simulink model "sim_FullMRE_case5"  (R2023a)
settings: Solver=ode3  StartTime=0.0  StopTime=500  FixedStep=Ts  MaxStep=Ts  RelTol=1e-4
values from neighbouring files (symbols this model uses):
  b0 = 30    [Initial_par.m]    (also in Test_par.m)
  b1 = 11    [Initial_par.m]    (also in Test_par.m)
  c1 = 1/5    (= 0.2)    [Initial_par.m]    (also in Test_par.m = 1)
  c2 = 1/5    (= 0.2)    [Initial_par.m]    (also in Test_par.m = 1)
  c3 = 1/5    (= 0.2)    [Initial_par.m]    (also in Test_par.m = 1)
  gamma = 20    [Initial_par.m]    (also in Test_par.m = 1)
  kpa = [kap1,kap2,kap3]    [Initial_par.m]    (also in Test_par.m)
  N = 3    [Initial_par.m]    (also in Test_par.m)
  p0 = 625    [Initial_par.m]    (also in Test_par.m = 10000)
  p1 = 500    [Initial_par.m]    (also in Test_par.m = 4000)
  p2 = 150    [Initial_par.m]    (also in Test_par.m = 600)
  p3 = 20    [Initial_par.m]    (also in Test_par.m = 40)
  th = [0.1,0.5,1.5]'    [Initial_par.m]    (also in Test_par.m = [0.4,0.5,0.1]')
  Ts = 1e-3    (= 0.001)    [Initial_par.m]    (also in Test_par.m; fig_test_draw.m)
  vari = SD^2    (= 1e-06)    [Initial_par.m]    (also in Test_par.m)
  x0 = [0,0,0]'    [Initial_par.m]    (also in TO_sys.m = x_init; Test_par.m)
  zeta0 = -z0    [Initial_par.m]    (also in Test_par.m)
undefined symbols (not defined in the file or in its folder): Phi0, z0
libraries: matrix_library x5
settings Model: Creator=stt  LastModifiedBy=stt
settings SolverCC: SolverResetMethod=Robust
settings OptimizationCC: ReuseModelBlockBuffer=off

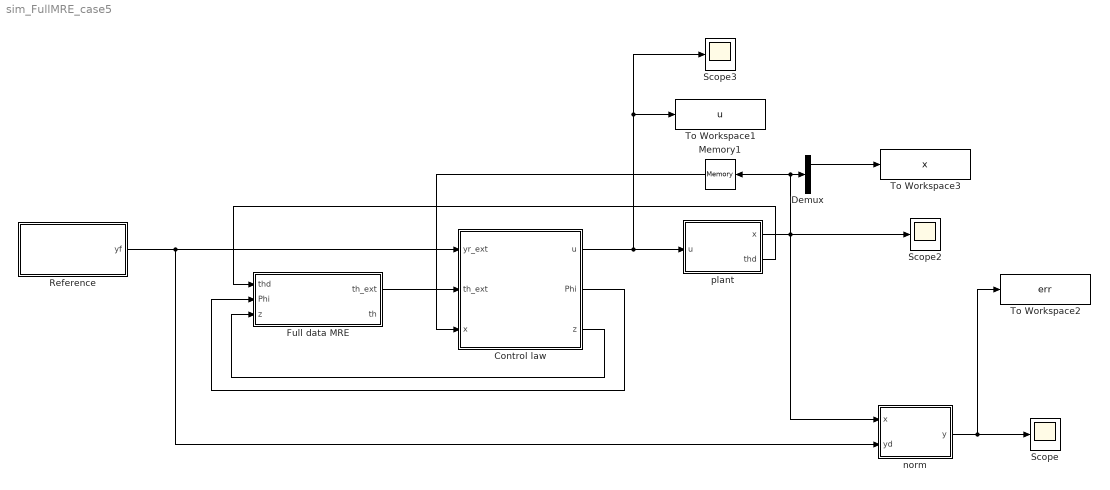
== system sim_FullMRE_case5 ==
  Control law : Subsystem
  Demux : Demux  Outputs=3
  Full data MRE : Subsystem
  Memory1 : Memory  InitialCondition=x0
  Reference : Subsystem
  Scope : Scope
  Scope2 : Scope
  Scope3 : Scope
  To Workspace1 : ToWorkspace  VariableName=u  SaveFormat=Timeseries  SampleTime=-1
  To Workspace2 : ToWorkspace  VariableName=err  SaveFormat=Timeseries  SampleTime=-1
  To Workspace3 : ToWorkspace  VariableName=x  SaveFormat=Timeseries  SampleTime=-1
  norm : MATLAB Function  TreatAsAtomicUnit=on
  plant : Subsystem
  wires:
  norm/1(y) -> To Workspace2/1, Scope/1
  plant/1(x) -> Demux/1, Memory1/1, norm/1(x), Scope2/1
  Demux/1 -> To Workspace3/1
  Control law/2(Phi) -> Full data MRE/2(Phi)
  Control law/1(u) -> To Workspace1/1, Scope3/1, plant/1(u)
  Memory1/1 -> Control law/3(x)
  Full data MRE/1(th_ext) -> Control law/2(th_ext)
  Control law/3(z) -> Full data MRE/3(z)
  plant/2(thd) -> Full data MRE/1(thd)
  Reference/1(yf) -> norm/2(yd), Control law/1(yr_ext)

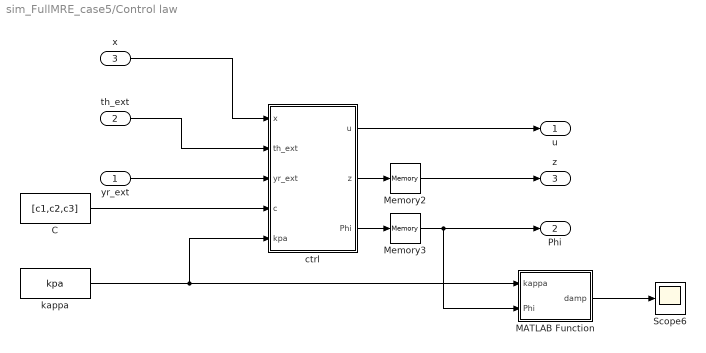
== system sim_FullMRE_case5/Control law ==
  yr_ext : Inport
  th_ext : Inport  Port=2
  x : Inport  Port=3
  C : Constant  Value=[c1,c2,c3]
  MATLAB Function : MATLAB Function  TreatAsAtomicUnit=on
  Memory2 : Memory  InitialCondition=z0
  Memory3 : Memory  InitialCondition=Phi0
  Scope6 : Scope
  ctrl : MATLAB Function  TreatAsAtomicUnit=on
  kappa : Constant  Value=kpa
  u : Outport
  Phi : Outport  Port=2
  z : Outport  Port=3
  wires:
  ctrl/3(Phi) -> Memory3/1
  Memory3/1 -> MATLAB Function/2(Phi), Phi/1
  th_ext/1 -> ctrl/2(th_ext)
  kappa/1 -> ctrl/5(kpa), MATLAB Function/1(kappa)
  C/1 -> ctrl/4(c)
  Memory2/1 -> z/1
  ctrl/2(z) -> Memory2/1
  yr_ext/1 -> ctrl/3(yr_ext)
  x/1 -> ctrl/1(x)
  ctrl/1(u) -> u/1
  MATLAB Function/1(damp) -> Scope6/1

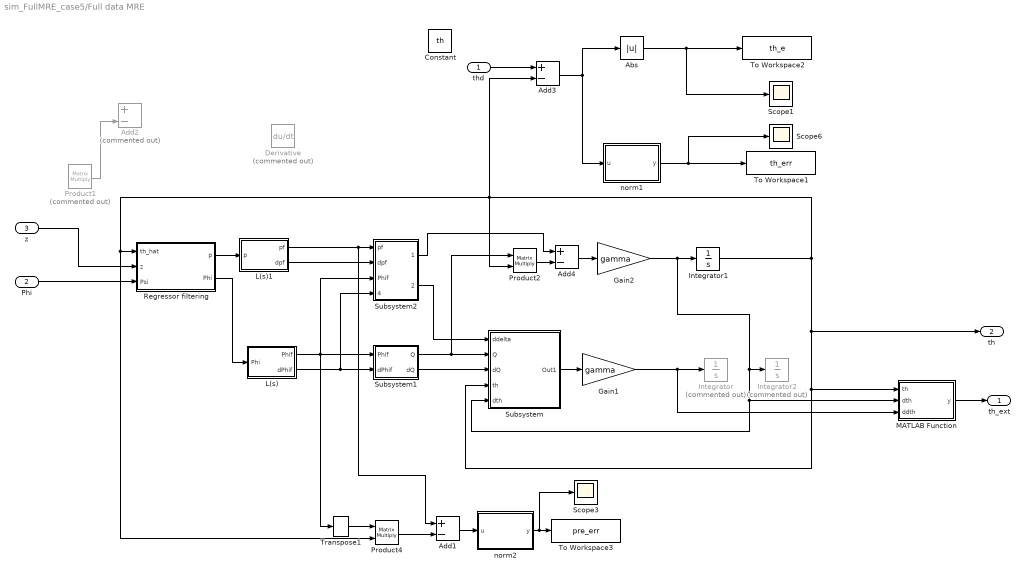
== system sim_FullMRE_case5/Full data MRE ==
  thd : Inport
  Phi : Inport  Port=2
  z : Inport  Port=3
  Abs : Abs  SaturateOnIntegerOverflow=off
  Add1 : Sum  Inputs=+-
  Add2 : Sum  Commented=on  Inputs=+-
  Add3 : Sum  Inputs=+-
  Add4 : Sum  Inputs=+-
  Constant : Constant  Value=th
  Derivative : Derivative  Commented=on
  Gain1 : Gain  Gain=gamma
  Gain2 : Gain  Gain=gamma
  Integrator : Integrator  Commented=on  InitialCondition=zeros(N,1)
  Integrator1 : Integrator  InitialCondition=zeros(N,1)
  Integrator2 : Integrator  Commented=on  InitialCondition=zeros(N,1)
  L(s) : Subsystem
  L(s)1 : Subsystem
  MATLAB Function : MATLAB Function  TreatAsAtomicUnit=on
  Product1 : Product  Commented=on  Multiplication=Matrix(*)
  Product2 : Product  Multiplication=Matrix(*)
  Product4 : Product  Multiplication=Matrix(*)
  Regressor filtering : Subsystem
  Scope1 : Scope
  Scope3 : Scope
  Scope6 : Scope
  Subsystem : Subsystem
  Subsystem1 : Subsystem
  Subsystem2 : Subsystem
  To Workspace1 : ToWorkspace  VariableName=th_err  SaveFormat=Timeseries  SampleTime=-1
  To Workspace2 : ToWorkspace  VariableName=th_e  SaveFormat=Timeseries  SampleTime=-1
  To Workspace3 : ToWorkspace  VariableName=pre_err  SaveFormat=Timeseries  SampleTime=-1
  Transpose1 : matrix_library/Transpose
  norm1 : MATLAB Function  TreatAsAtomicUnit=on
  norm2 : MATLAB Function  TreatAsAtomicUnit=on
  th_ext : Outport
  th : Outport  Port=2
  wires:
  MATLAB Function/1(y) -> th_ext/1
  norm1/1(y) -> To Workspace1/1, Scope6/1
  thd/1 -> Add3/1
  Regressor filtering/2(Phi) -> L(s)/1(Phi)
  Regressor filtering/1(p) -> L(s)1/1(p)
  z/1 -> Regressor filtering/2(z)
  Phi/1 -> Regressor filtering/3(Psi)
  L(s)/1(Phif) -> Subsystem2/3(Phif), Transpose1/1, Subsystem1/1(Phif)
  L(s)/2(dPhif) -> Subsystem2/4(dPhif), Subsystem1/2(dPhif)
  Integrator1/1 -> Subsystem/4(th), MATLAB Function/1(th), th/1, Add3/2, Product2/2, Product4/2, Regressor filtering/1(th_hat)
  L(s)1/2(dpf) -> Subsystem2/2(dpf)
  Subsystem1/1(Q) -> Product2/1, Subsystem/2(Q)
  Add3/1 -> norm1/1(u), Abs/1
  Abs/1 -> To Workspace2/1, Scope1/1
  norm2/1(y) -> Scope3/1, To Workspace3/1
  Add1/1 -> norm2/1(u)
  Product4/1 -> Add1/2
  Transpose1/1 -> Product4/1
  L(s)1/1(pf) -> Add1/1, Subsystem2/1(pf)
  Subsystem/1(Out1) -> Gain1/1
  Product1/1 -> Add2/2
  Subsystem1/2(dQ) -> Subsystem/3(dQ)
  Subsystem2/2(ddelta) -> Subsystem/1(ddelta)
  Gain1/1 -> MATLAB Function/3(ddth), Integrator/1
  Gain2/1 -> Integrator2/1, MATLAB Function/2(dth), Subsystem/5(dth), Integrator1/1
  Product2/1 -> Add4/2
  Subsystem2/1(delta) -> Add4/1
  Add4/1 -> Gain2/1

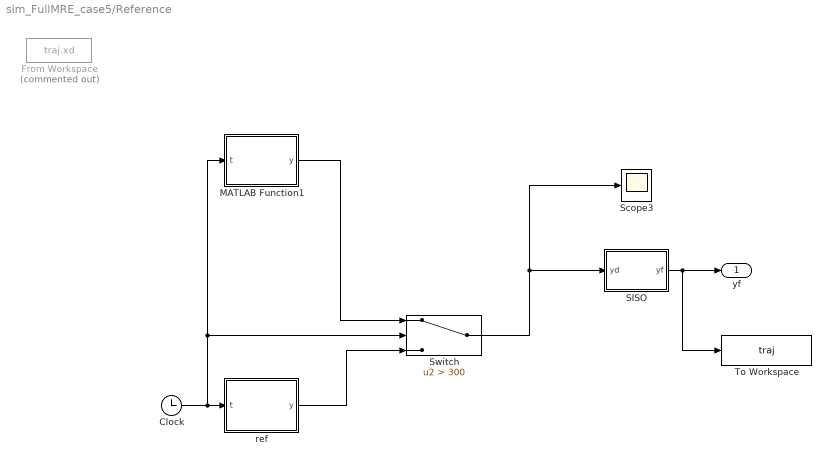
== system sim_FullMRE_case5/Reference ==
  Clock : Clock
  From Workspace : FromWorkspace  Commented=on  VariableName=traj.xd
  MATLAB Function1 : MATLAB Function  TreatAsAtomicUnit=on
  SISO : Subsystem
  Scope3 : Scope
  Switch : Switch  Criteria=u2 > Threshold  Threshold=300  SaturateOnIntegerOverflow=off  InputSameDT=off
  To Workspace : ToWorkspace  VariableName=traj  SaveFormat=Timeseries  SampleTime=-1
  ref : MATLAB Function  TreatAsAtomicUnit=on
  yf : Outport
  wires:
  Switch/1 -> Scope3/1, SISO/1(yd)
  Clock/1 -> MATLAB Function1/1(t), Switch/2, ref/1(t)
  ref/1(y) -> Switch/3
  MATLAB Function1/1(y) -> Switch/1
  SISO/1(yf) -> To Workspace/1, yf/1

== system sim_FullMRE_case5/plant ==
  u : Inport
  Add : Sum
  MATLAB Function : MATLAB Function  TreatAsAtomicUnit=on
  Random Number : RandomNumber  Variance=vari  SampleTime=Ts
  S-Function : S-Function  FunctionName=TO_sys  Parameters=x0,th  SFunctionDeploymentMode=off  EnableBusSupport=off
  x : Outport
  thd : Outport  Port=2
  wires:
  u/1 -> S-Function/1
  S-Function/1 -> MATLAB Function/1(u)
  Add/1 -> x/1
  MATLAB Function/2(thd) -> thd/1
  MATLAB Function/1(x) -> Add/2
  Random Number/1 -> Add/1

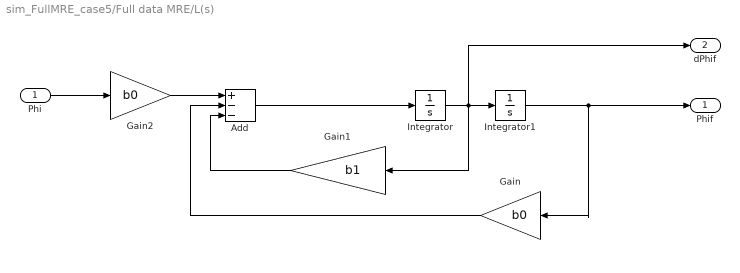
== system sim_FullMRE_case5/Full data MRE/L(s) ==
  Phi : Inport
  Add : Sum  Inputs=+--
  Gain : Gain  Gain=b0
  Gain1 : Gain  Gain=b1
  Gain2 : Gain  Gain=b0
  Integrator : Integrator
  Integrator1 : Integrator
  Phif : Outport
  dPhif : Outport  Port=2
  wires:
  Phi/1 -> Gain2/1
  Integrator1/1 -> Gain/1, Phif/1
  Add/1 -> Integrator/1
  Integrator/1 -> Gain1/1, dPhif/1, Integrator1/1
  Gain1/1 -> Add/3
  Gain/1 -> Add/2
  Gain2/1 -> Add/1

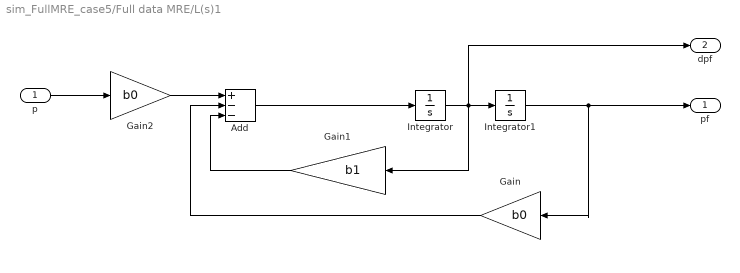
== system sim_FullMRE_case5/Full data MRE/L(s)1 ==
  p : Inport
  Add : Sum  Inputs=+--
  Gain : Gain  Gain=b0
  Gain1 : Gain  Gain=b1
  Gain2 : Gain  Gain=b0
  Integrator : Integrator
  Integrator1 : Integrator
  pf : Outport
  dpf : Outport  Port=2
  wires:
  p/1 -> Gain2/1
  Integrator1/1 -> Gain/1, pf/1
  Add/1 -> Integrator/1
  Integrator/1 -> Gain1/1, dpf/1, Integrator1/1
  Gain1/1 -> Add/3
  Gain/1 -> Add/2
  Gain2/1 -> Add/1

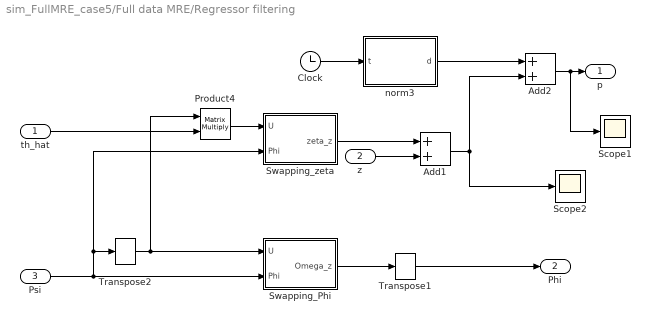
== system sim_FullMRE_case5/Full data MRE/Regressor filtering ==
  th_hat : Inport
  z : Inport  Port=2
  Psi : Inport  Port=3
  Add1 : Sum
  Add2 : Sum
  Clock : Clock
  Product4 : Product  Multiplication=Matrix(*)
  Scope1 : Scope
  Scope2 : Scope
  Swapping_Phi : Subsystem
  Swapping_zeta : Subsystem
  Transpose1 : matrix_library/Transpose
  Transpose2 : matrix_library/Transpose
  norm3 : MATLAB Function  TreatAsAtomicUnit=on
  p : Outport
  Phi : Outport  Port=2
  wires:
  Product4/1 -> Swapping_zeta/1(U)
  th_hat/1 -> Product4/2
  Psi/1 -> Swapping_Phi/2(Phi), Swapping_zeta/2(Phi), Transpose2/1
  Swapping_zeta/1(zeta_z) -> Add1/1
  Transpose2/1 -> Swapping_Phi/1(U), Product4/1
  z/1 -> Add1/2
  Add1/1 -> Add2/2, Scope2/1
  Swapping_Phi/1(Omega_z) -> Transpose1/1
  Transpose1/1 -> Phi/1
  Clock/1 -> norm3/1(t)
  Add2/1 -> Scope1/1, p/1
  norm3/1(d) -> Add2/1

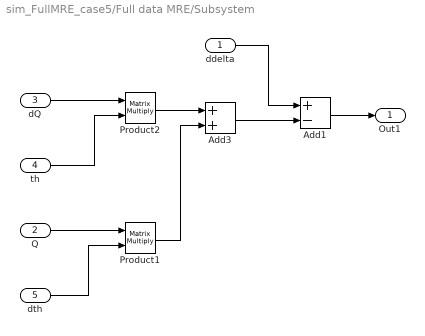
== system sim_FullMRE_case5/Full data MRE/Subsystem ==
  ddelta : Inport
  Q : Inport  Port=2
  dQ : Inport  Port=3
  th : Inport  Port=4
  dth : Inport  Port=5
  Add1 : Sum  Inputs=+-
  Add3 : Sum
  Product1 : Product  Multiplication=Matrix(*)
  Product2 : Product  Multiplication=Matrix(*)
  Out1 : Outport
  wires:
  dQ/1 -> Product2/1
  th/1 -> Product2/2
  Product2/1 -> Add3/1
  Q/1 -> Product1/1
  dth/1 -> Product1/2
  Product1/1 -> Add3/2
  Add3/1 -> Add1/2
  ddelta/1 -> Add1/1
  Add1/1 -> Out1/1

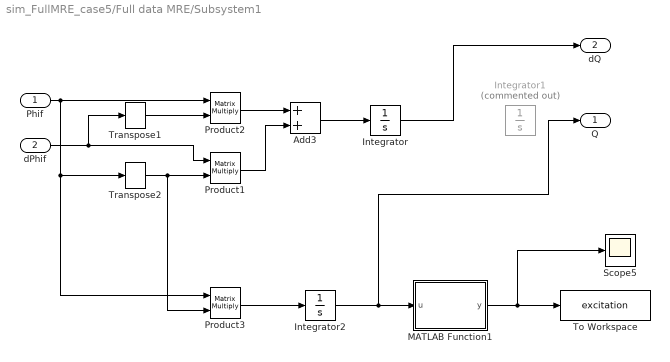
== system sim_FullMRE_case5/Full data MRE/Subsystem1 ==
  Phif : Inport
  dPhif : Inport  Port=2
  Add3 : Sum
  Integrator : Integrator
  Integrator1 : Integrator  Commented=on
  Integrator2 : Integrator
  MATLAB Function1 : MATLAB Function  TreatAsAtomicUnit=on
  Product1 : Product  Multiplication=Matrix(*)
  Product2 : Product  Multiplication=Matrix(*)
  Product3 : Product  Multiplication=Matrix(*)
  Scope5 : Scope
  To Workspace : ToWorkspace  VariableName=excitation  SaveFormat=Timeseries  SampleTime=-1
  Transpose1 : matrix_library/Transpose
  Transpose2 : matrix_library/Transpose
  Q : Outport
  dQ : Outport  Port=2
  wires:
  Phif/1 -> Product2/1, Product3/1, Transpose2/1
  dPhif/1 -> Product1/1, Transpose1/1
  Product1/1 -> Add3/2
  Transpose1/1 -> Product2/2
  Transpose2/1 -> Product3/2, Product1/2
  Product2/1 -> Add3/1
  Add3/1 -> Integrator/1
  Integrator/1 -> dQ/1
  Integrator2/1 -> Q/1, MATLAB Function1/1(u)
  Product3/1 -> Integrator2/1
  MATLAB Function1/1(y) -> Scope5/1, To Workspace/1

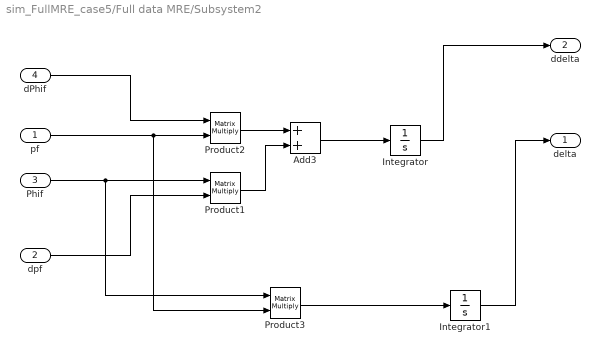
== system sim_FullMRE_case5/Full data MRE/Subsystem2 ==
  pf : Inport
  dpf : Inport  Port=2
  Phif : Inport  Port=3
  dPhif : Inport  Port=4
  Add3 : Sum
  Integrator : Integrator
  Integrator1 : Integrator
  Product1 : Product  Multiplication=Matrix(*)
  Product2 : Product  Multiplication=Matrix(*)
  Product3 : Product  Multiplication=Matrix(*)
  delta : Outport
  ddelta : Outport  Port=2
  wires:
  Product1/1 -> Add3/2
  Product2/1 -> Add3/1
  Integrator/1 -> ddelta/1
  Integrator1/1 -> delta/1
  pf/1 -> Product3/2, Product2/2
  dPhif/1 -> Product2/1
  Phif/1 -> Product3/1, Product1/1
  dpf/1 -> Product1/2
  Add3/1 -> Integrator/1
  Product3/1 -> Integrator1/1

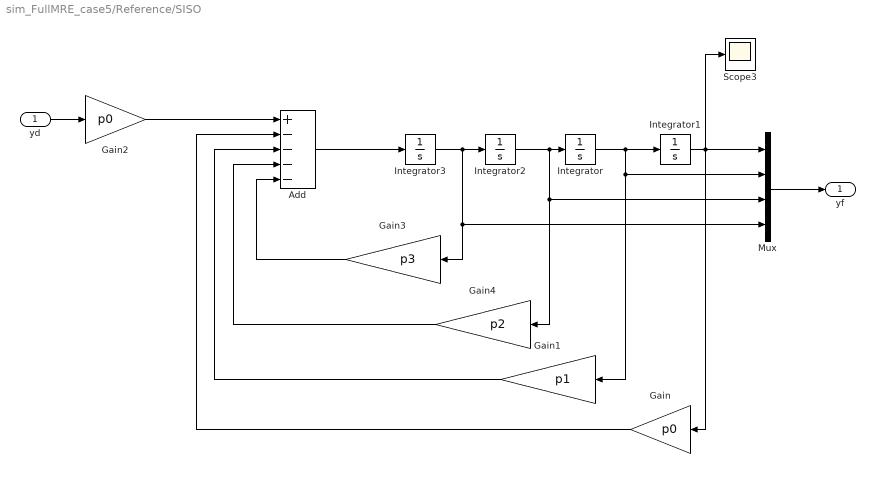
== system sim_FullMRE_case5/Reference/SISO ==
  yd : Inport
  Add : Sum  Inputs=+----
  Gain : Gain  Gain=p0
  Gain1 : Gain  Gain=p1
  Gain2 : Gain  Gain=p0
  Gain3 : Gain  Gain=p3
  Gain4 : Gain  Gain=p2
  Integrator{,1..3} (4 alike) : Integrator
  Mux : Mux
  Scope3 : Scope
  yf : Outport
  wires:
  yd/1 -> Gain2/1
  Add/1 -> Integrator3/1
  Integrator/1 -> Gain1/1, Mux/2, Integrator1/1
  Gain1/1 -> Add/3
  Gain/1 -> Add/2
  Gain2/1 -> Add/1
  Integrator2/1 -> Gain4/1, Mux/3, Integrator/1
  Integrator3/1 -> Gain3/1, Mux/4, Integrator2/1
  Gain3/1 -> Add/5
  Gain4/1 -> Add/4
  Mux/1 -> yf/1
  Integrator1/1 -> Mux/1, Scope3/1, Gain/1

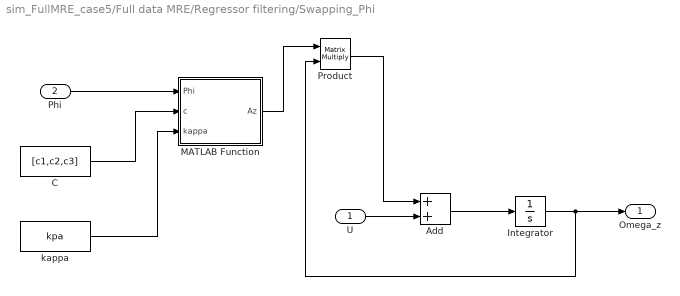
== system sim_FullMRE_case5/Full data MRE/Regressor filtering/Swapping_Phi ==
  U : Inport
  Phi : Inport  Port=2
  Add : Sum
  C : Constant  Value=[c1,c2,c3]
  Integrator : Integrator
  MATLAB Function : MATLAB Function  TreatAsAtomicUnit=on
  Product : Product  Multiplication=Matrix(*)
  kappa : Constant  Value=kpa
  Omega_z : Outport
  wires:
  Phi/1 -> MATLAB Function/1(Phi)
  C/1 -> MATLAB Function/2(c)
  kappa/1 -> MATLAB Function/3(kappa)
  MATLAB Function/1(Az) -> Product/1
  Product/1 -> Add/1
  Add/1 -> Integrator/1
  U/1 -> Add/2
  Integrator/1 -> Product/2, Omega_z/1

== system sim_FullMRE_case5/Full data MRE/Regressor filtering/Swapping_zeta ==
  U : Inport
  Phi : Inport  Port=2
  Add : Sum
  C : Constant  Value=[c1,c2,c3]
  Integrator : Integrator  InitialCondition=zeta0
  MATLAB Function : MATLAB Function  TreatAsAtomicUnit=on
  Product : Product  Multiplication=Matrix(*)
  kappa : Constant  Value=kpa
  zeta_z : Outport
  wires:
  Phi/1 -> MATLAB Function/1(Phi)
  C/1 -> MATLAB Function/2(c)
  kappa/1 -> MATLAB Function/3(kappa)
  MATLAB Function/1(Az) -> Product/1
  Product/1 -> Add/1
  Add/1 -> Integrator/1
  U/1 -> Add/2
  Integrator/1 -> Product/2, zeta_z/1

== matlab function sim_FullMRE_case5/Full data MRE/norm2 ==
  data: u input; y output
function y = fcn(u)

y = norm(u);

== matlab function sim_FullMRE_case5/Control law/MATLAB Function ==
  data: kappa input; damp output; Phi input
function damp = fcn(kappa,Phi)
kap1=kappa(1);kap2=kappa(2);kap3=kappa(3);
phi1=Phi(:,1);phi2=Phi(:,2);phi3=Phi(:,3);
damp=-[kap1*norm(phi1)^2,kap2*norm(phi2)^2,kap3*norm(phi3)^2];

== matlab function sim_FullMRE_case5/Reference/ref ==
  data: t input; y output
function y = fcn(t)


if t<20
    y=0.6;
elseif t<60
    y=0.1;% - 0.4*(tanh((t-30)/5)-1)/2;
elseif t<100
    y=-0.4;% - 0.3*(tanh((t-80)/5)-1)/2;
else
    y=-0.2;
end
% if t<20
%     y=0.5+0.5*(tanh((t-10)/5)-1)/2;
% elseif t<60
%     y=0.3 - 0.2*(tanh((t-40)/5)-1)/2;
% elseif t<120
%     y=-0.2 - 0.5*(tanh((t-90)/5)-1)/2;
% else
%     y=-0.2; %- 0.9*(tanh((t-150)/5)-1)/2;
% end
% y=y*2;
% T=25;
% y=0.5*sin(t*2*pi/T);

% if t>=120
%     y=0;
% end

== matlab function sim_FullMRE_case5/Control law/ctrl ==
  data: x input; th_ext input; yr_ext input; u output; c input; kpa input; z output; Phi output
function [u,z,Phi] = fcn(x,th_ext,yr_ext,c,kpa)



[alpha1,alpha2,u,z,Phi]=virtual_ctrl(x,th_ext,yr_ext,kpa,c);
vir_u=[alpha1,alpha2];

== matlab function sim_FullMRE_case5/Full data MRE/Subsystem1/MATLAB Function1 ==
  data: u input; y output
function y = fcn(u)

y = min(svd(u));

== matlab function sim_FullMRE_case5/Reference/MATLAB Function1 ==
  data: y output; t input
function y = fcn(t)

T=25;

if t<300
    
    y=-0.2;
elseif t<400
    y=-0.2+0.1*sin((t-300)*2*pi/T);
else
    y=-0.2;
end

== matlab function sim_FullMRE_case5/norm ==
  data: x input; y output; yd input
function y= fcn(x,yd)
err=x(1)-yd(1);
y = abs(err);

== matlab function sim_FullMRE_case5/Full data MRE/Regressor filtering/Swapping_zeta/MATLAB Function ==
  data: Phi input; Az output; c input; kappa input
function Az = fcn(Phi,c,kappa)
c1=c(1);c2=c(2);c3=c(3);
kap1=kappa(1);kap2=kappa(2);kap3=kappa(3);
phi1=Phi(:,1);phi2=Phi(:,2);phi3=Phi(:,3);
Dg=-[c1+kap1*norm(phi1)^2,c2+kap2*norm(phi2)^2,c3+kap3*norm(phi3)^2];
Az=diag(Dg)+diag([1,1],1)-diag([1,1],-1);

== matlab function sim_FullMRE_case5/Full data MRE/Regressor filtering/Swapping_Phi/MATLAB Function ==
  data: Phi input; Az output; c input; kappa input
function Az = fcn(Phi,c,kappa)
c1=c(1);c2=c(2);c3=c(3);
kap1=kappa(1);kap2=kappa(2);kap3=kappa(3);
phi1=Phi(:,1);phi2=Phi(:,2);phi3=Phi(:,3);
Dg=-[c1+kap1*norm(phi1)^2,c2+kap2*norm(phi2)^2,c3+kap3*norm(phi3)^2];
Az=diag(Dg)+diag([1,1],1)-diag([1,1],-1);

== matlab function sim_FullMRE_case5/plant/MATLAB Function ==
  data: u input; x output; thd output
function [x,thd] = fcn(u)

x=u(1:3);
thd=u(4:6);

== matlab function sim_FullMRE_case5/Full data MRE/MATLAB Function ==
  data: th input; y output; dth input; ddth input
function y = fcn(th,dth,ddth)

y = [th,dth,ddth];

== matlab function sim_FullMRE_case5/Full data MRE/norm1 ==
  data: u input; y output
function y = fcn(u)

y = norm(u);

== matlab function sim_FullMRE_case5/Full data MRE/Regressor filtering/norm3 ==
  data: t input; d output
function d = fcn(t)

d = 0.015+0.005*sin(pi*t/5);%+0.005;
